simulink subsystem "ElectricalSystem2EMHev"  (R2022b)
settings: Solver=VariableStepAuto  StartTime=0.0  StopTime=10.0  RelTol=1e-3
settings Model: ModifiedByFormat=The MathWorks, Inc.  Creator=The MathWorks, Inc.  LastModifiedBy=The MathWorks, Inc.
settings SolverCC: MaxZcPerStep=1
settings DebuggingCC: UnconnectedInputMsg=warning  UnconnectedOutputMsg=warning  UnconnectedLineMsg=warning
settings ModelReferenceCC: EnableRefExpFcnMdlSchedulingChecks=on
settings RTWCC: DLArmComputeVersion=19.05

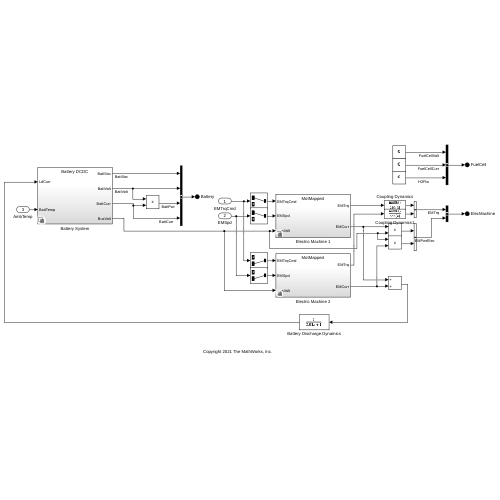
[thumbnail: Simulink's stored preview of the top-level diagram]
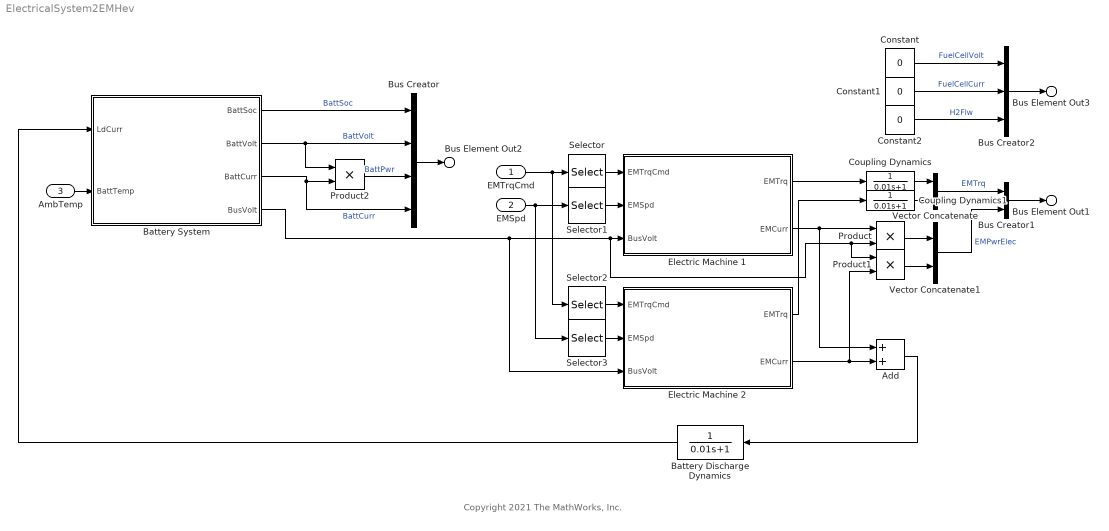
== system ElectricalSystem2EMHev ==
  note: Copyright 2021 The MathWorks, Inc.
  EMTrqCmd : Inport
  EMSpd : Inport  Port=2
  AmbTemp : Inport  Port=3
  Add : Sum
  Battery Discharge Dynamics : TransferFcn  Denominator=[0.01 1]
  Battery System : Subsystem  Variant=on  VariantControlMode=label  LabelModeActiveChoice=1
  Bus Creator : BusCreator  Inputs=4
  Bus Creator1 : BusCreator  Inputs=2
  Bus Creator2 : BusCreator  Inputs=3
  Constant : Constant  Value=0  SampleTime=-1
  Constant1 : Constant  Value=0  SampleTime=-1
  Constant2 : Constant  Value=0  SampleTime=-1
  Coupling Dynamics : TransferFcn  Denominator=[0.01 1]
  Coupling Dynamics1 : TransferFcn  Denominator=[0.01 1]
  Electric Machine 1 : Subsystem  Variant=on  VariantControlMode=label  LabelModeActiveChoice=0
  Electric Machine 2 : Subsystem  Variant=on  VariantControlMode=label  LabelModeActiveChoice=0
  Product : Product
  Product1 : Product
  Product2 : Product
  Selector : Selector  InputPortWidth=2  IndexOptions=Index vector (dialog)  Indices=[1]  OutputSizes=1
  Selector1 : Selector  InputPortWidth=2  IndexOptions=Index vector (dialog)  Indices=[1]  OutputSizes=1
  Selector2 : Selector  InputPortWidth=2  IndexOptions=Index vector (dialog)  Indices=[2]  OutputSizes=1
  Selector3 : Selector  InputPortWidth=2  IndexOptions=Index vector (dialog)  Indices=[2]  OutputSizes=1
  Vector Concatenate : Concatenate
  Vector Concatenate1 : Concatenate
  Bus Element Out2 : Outport  PortName=Battery
  Bus Element Out1 : Outport  Port=2  PortName=ElecMachine
  Bus Element Out3 : Outport  Port=3  PortName=FuelCell
  wires:
  Bus Creator2/1 -> Bus Element Out3/1
  Constant2/1 -> Bus Creator2/3  "H2Flw"
  Constant/1 -> Bus Creator2/1  "FuelCellVolt"
  Constant1/1 -> Bus Creator2/2  "FuelCellCurr"
  Bus Creator1/1 -> Bus Element Out1/1
  Bus Creator/1 -> Bus Element Out2/1
  Coupling Dynamics/1 -> Vector Concatenate/1
  Coupling Dynamics1/1 -> Vector Concatenate/2
  Vector Concatenate/1 -> Bus Creator1/1  "EMTrq"
  Product1/1 -> Vector Concatenate1/2
  Product/1 -> Vector Concatenate1/1
  Vector Concatenate1/1 -> Bus Creator1/2  "EMPwrElec"
  Selector3/1 -> Electric Machine 2/2(EMSpd)
  Selector2/1 -> Electric Machine 2/1(EMTrqCmd)
  Selector1/1 -> Electric Machine 1/2(EMSpd)
  Selector/1 -> Electric Machine 1/1(EMTrqCmd)
  Electric Machine 2/1(EMTrq) -> Coupling Dynamics1/1
  Add/1 -> Battery Discharge Dynamics/1
  Electric Machine 2/2(EMCurr) -> Product1/2, Add/2
  Battery System/2(BattVolt) -> Product2/1, Bus Creator/2  "BattVolt"
  EMTrqCmd/1 -> Selector/1, Selector2/1
  Battery System/1(BattSoc) -> Bus Creator/1  "BattSoc"
  EMSpd/1 -> Selector1/1, Selector3/1
  Battery System/4(BusVolt) -> Electric Machine 2/3(BusVolt), Product1/1, Product/2, Electric Machine 1/3(BusVolt)
  Battery System/3(BattCurr) -> Bus Creator/4, Product2/2  "BattCurr"
  AmbTemp/1 -> Battery System/2(BattTemp)
  Product2/1 -> Bus Creator/3  "BattPwr"
  Battery Discharge Dynamics/1 -> Battery System/1(LdCurr)
  Electric Machine 1/1(EMTrq) -> Coupling Dynamics/1
  Electric Machine 1/2(EMCurr) -> Add/1, Product/1

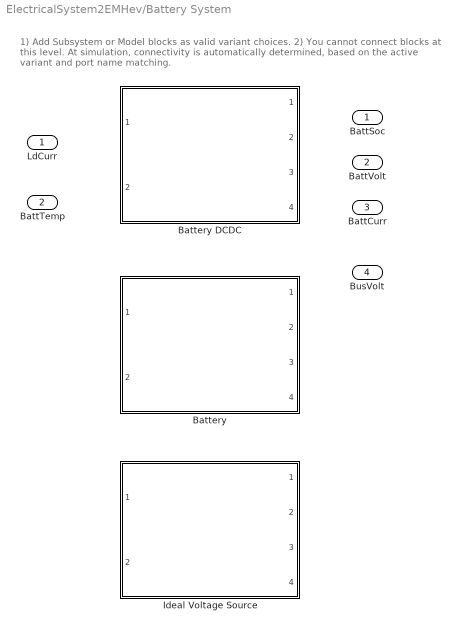
== system ElectricalSystem2EMHev/Battery System ==
  note: 1) Add Subsystem or Model blocks as valid variant choices.
      | 2) You cannot connect blocks at this level. At simulation, connectivity is automatically
      | determined, based on the active variant and port name matching.
  LdCurr : Inport
  BattTemp : Inport  Port=2
  Battery : Subsystem  VariantControl=0  ReferencedSubsystem=Battery
  Battery DCDC : Subsystem  VariantControl=1  ReferencedSubsystem=BatteryDCDC
  Ideal Voltage Source : Subsystem  VariantControl=2  ReferencedSubsystem=IdealVoltageSource
  BattSoc : Outport  VectorParamsAs1DForOutWhenUnconnected=off
  BattVolt : Outport  Port=2  VectorParamsAs1DForOutWhenUnconnected=off
  BattCurr : Outport  Port=3  VectorParamsAs1DForOutWhenUnconnected=off
  BusVolt : Outport  Port=4  VectorParamsAs1DForOutWhenUnconnected=off

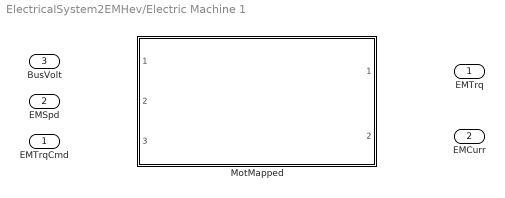
== system ElectricalSystem2EMHev/Electric Machine 1 ==
  EMTrqCmd : Inport
  EMSpd : Inport  Port=2
  BusVolt : Inport  Port=3
  MotMapped : Subsystem  VariantControl=0  ReferencedSubsystem=ElectricMachine1
  EMTrq : Outport  VectorParamsAs1DForOutWhenUnconnected=off
  EMCurr : Outport  Port=2  VectorParamsAs1DForOutWhenUnconnected=off

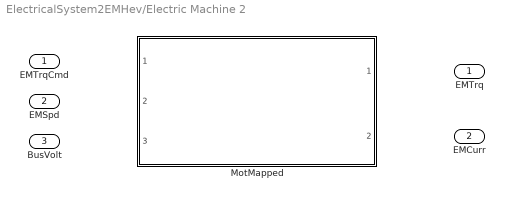
== system ElectricalSystem2EMHev/Electric Machine 2 ==
  EMTrqCmd : Inport
  EMSpd : Inport  Port=2
  BusVolt : Inport  Port=3
  MotMapped : Subsystem  VariantControl=0  ReferencedSubsystem=ElectricMachine2
  EMTrq : Outport  VectorParamsAs1DForOutWhenUnconnected=off
  EMCurr : Outport  Port=2  VectorParamsAs1DForOutWhenUnconnected=off
